simulink model "AM"  (R2018a)
settings: Solver=VariableStepAuto  StartTime=0.0  StopTime=10.0  RelTol=1e-3
libraries: dspfdesign x1
settings Model: Creator=BlueFlash  LastModifiedBy=BlueFlash

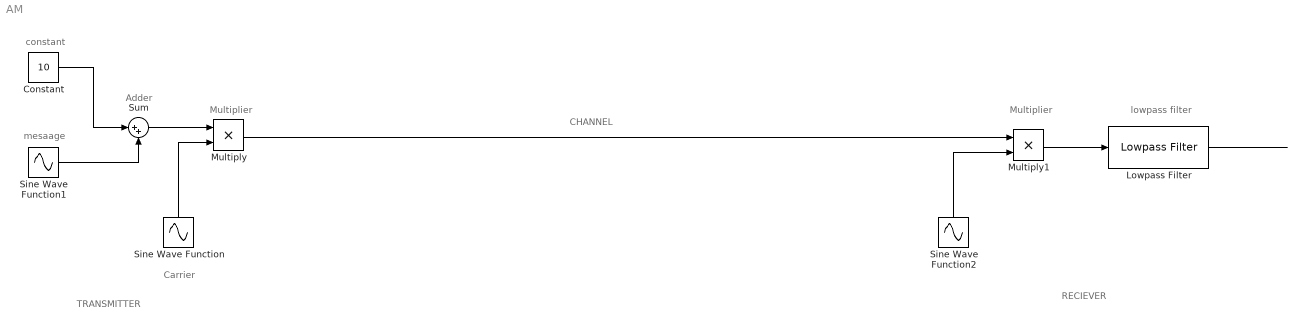
== system AM ==
  note: RECIEVER
  note: TRANSMITTER
  note: lowpass filter
  note: CHANNEL
  note: Multiplier
  note: Adder
  note: constant
  note: Carrier
  note: mesaage
  note: Multiplier
  Constant : Constant  Value=10
  Lowpass Filter : dspfdesign/Lowpass Filter  FilterType=FIR  DesignForMinimumOrder=on  FilterOrder=50  PassbandFrequency=100  StopbandFrequency=1000  PassbandRipple=0.1  StopbandAttenuation=80  InheritSampleRate=off  SampleRate=44100  SimulateUsing=Interpreted execution  roundingMode=Floor  coeffsDataTypeStr=fixdt(1,16)
  Multiply : Product
  Multiply1 : Product
  Sine Wave Function : Sin  Amplitude=10  Frequency=1000  SampleTime=0.0001
  Sine Wave Function1 : Sin  Amplitude=5  Frequency=100  SampleTime=0.0001
  Sine Wave Function2 : Sin  Amplitude=10  Frequency=1000  SampleTime=0.0001
  Sum : Sum  Inputs=|++
  wires:
  Sine Wave Function/1 -> Multiply/2
  Sum/1 -> Multiply/1
  Constant/1 -> Sum/1
  Sine Wave Function1/1 -> Sum/2
  Sine Wave Function2/1 -> Multiply1/2
  Multiply/1 -> Multiply1/1
  Multiply1/1 -> Lowpass Filter/1
  Lowpass Filter/1 -> ?
